simulink model "deltaL"  (R2018b)
settings: Solver=VariableStepAuto  StartTime=0.0  StopTime=10.0  RelTol=1e-3
undefined symbols (not defined in the file or in its folder): lx, ly, lz
libraries: vrlib x2
settings Model: Creator=Erin B  LastModifiedBy=Erin B

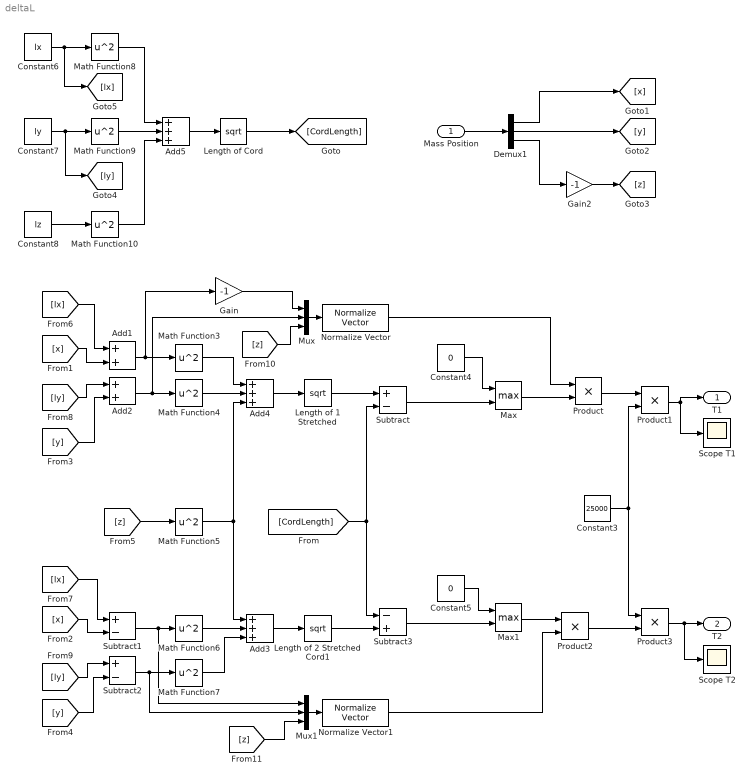
== system deltaL ==
  Mass Position : Inport
  Add1 : Sum
  Add2 : Sum
  Add3 : Sum  Inputs=+++
  Add4 : Sum  Inputs=+++
  Add5 : Sum  Inputs=+++
  Constant3 : Constant  Value=25000
  Constant4 : Constant  Value=0
  Constant5 : Constant  Value=0
  Constant6 : Constant  Value=lx
  Constant7 : Constant  Value=ly
  Constant8 : Constant  Value=lz
  Demux1 : Demux  Outputs=3
  Gain : Gain  Gain=-1
  Gain2 : Gain  Gain=-1
  Length of 1 Stretched : Sqrt  SaturateOnIntegerOverflow=on
  Length of 2 Stretched Cord1 : Sqrt  SaturateOnIntegerOverflow=on
  Length of Cord : Sqrt  SaturateOnIntegerOverflow=on
  Math Function{3..10} (8 alike) : Math  Operator=square  SaturateOnIntegerOverflow=on
  Max : MinMax  Function=max  Inputs=2
  Max1 : MinMax  Function=max  Inputs=2
  Mux : Mux  Inputs=3
  Mux1 : Mux  Inputs=3
  Normalize Vector : vrlib/Utilities/Normalize Vector  maxzero=0
      settings: SourceProductName=Simulink 3D Animation  SourceProductBaseCode=VR
  Normalize Vector1 : vrlib/Utilities/Normalize Vector  maxzero=0
      settings: SourceProductName=Simulink 3D Animation  SourceProductBaseCode=VR
  Product{,1..3} (4 alike) : Product
  Scope T1 : Scope
  Scope T2 : Scope
  Subtract : Sum  Inputs=+-
  Subtract1 : Sum  Inputs=+-
  Subtract2 : Sum  Inputs=+-
  Subtract3 : Sum  Inputs=-+
  T1 : Outport
  T2 : Outport  Port=2
  wires:
  Length of 1 Stretched/1 -> Subtract/1
  [lx] -> Subtract1/1
  [CordLength] -> Subtract/2, Subtract3/1
  [x] -> Add1/2
  [y] -> Add2/2
  Math Function4/1 -> Add4/2
  Math Function3/1 -> Add4/1
  Math Function5/1 -> Add4/3, Add3/1
  Add4/1 -> Length of 1 Stretched/1
  Add2/1 -> Mux/2, Math Function4/1
  Add1/1 -> Gain/1, Math Function3/1
  Mux/1 -> Normalize Vector/1
  Product2/1 -> Product3/2
  Constant4/1 -> Max/1
  Max/1 -> Product/2
  Constant3/1 -> Product1/2, Product3/1
  Product/1 -> Product1/1
  Subtract/1 -> Max/2
  Product3/1 -> Scope T2/1, T2/1
  Product1/1 -> Scope T1/1, T1/1
  Normalize Vector/1 -> Product/1
  Subtract2/1 -> Mux1/2, Math Function7/1
  Math Function6/1 -> Add3/2
  Math Function7/1 -> Add3/3
  Add3/1 -> Length of 2 Stretched Cord1/1
  Length of 2 Stretched Cord1/1 -> Subtract3/2
  Subtract3/1 -> Max1/2
  Constant5/1 -> Max1/1
  Mux1/1 -> Normalize Vector1/1
  Max1/1 -> Product2/1
  Normalize Vector1/1 -> Product2/2
  Subtract1/1 -> Mux1/1, Math Function6/1
  Gain/1 -> Mux/1
  [z] -> Math Function5/1
  Math Function8/1 -> Add5/1
  Add5/1 -> Length of Cord/1
  Constant7/1 -> [ly], Math Function9/1
  Math Function10/1 -> Add5/3
  Constant8/1 -> Math Function10/1
  Math Function9/1 -> Add5/2
  Constant6/1 -> [lx], Math Function8/1
  Length of Cord/1 -> [CordLength]
  Mass Position/1 -> Demux1/1
  Demux1/1 -> [x]
  [x] -> Subtract1/2
  Demux1/2 -> [y]
  [y] -> Subtract2/2
  Gain2/1 -> [z]
  Demux1/3 -> Gain2/1
  [lx] -> Add1/1
  [ly] -> Add2/1
  [ly] -> Subtract2/1
  [z] -> Mux/3
  [z] -> Mux1/3
